simulink model "mpcLKAsystem"  (R2020b)
settings: Solver=VariableStepAuto  StartTime=0.0  StopTime=15  RelTol=1e-3
values from neighbouring files (symbols this model uses):
  Cf = 19000    [VehicleSteeringControlExample.m]
  Cr = 33000    [VehicleSteeringControlExample.m]
  Iz = 2875    [VehicleSteeringControlExample.m]
  lf = 1.2    [VehicleSteeringControlExample.m]
  lr = 1.6    [VehicleSteeringControlExample.m]
  m = 1575    [VehicleSteeringControlExample.m]
  md = getCurvature(Vx,time)    [VehicleSteeringControlExample.m]
  Ts = 0.1    [VehicleSteeringControlExample.m]
  Vx = 15    [VehicleSteeringControlExample.m]
libraries: mpcadaslib x1
settings Model: Creator=The MathWorks, Inc.  LastModifiedBy=j10
settings DataIOCC: ReturnWorkspaceOutputs=off
settings DebuggingCC: ArithmeticOperatorsInVariantConditions=warning
settings SFSimCC: SimUseLocalCustomCode=off  CustomCodeUndefinedFunction=UseInterfaceOnly
settings RTWCC: RTWUseLocalCustomCode=off
settings CodeAppCC: StateflowObjectComments=on
settings SimscapeCC: SimscapeNormalizeSystem=off

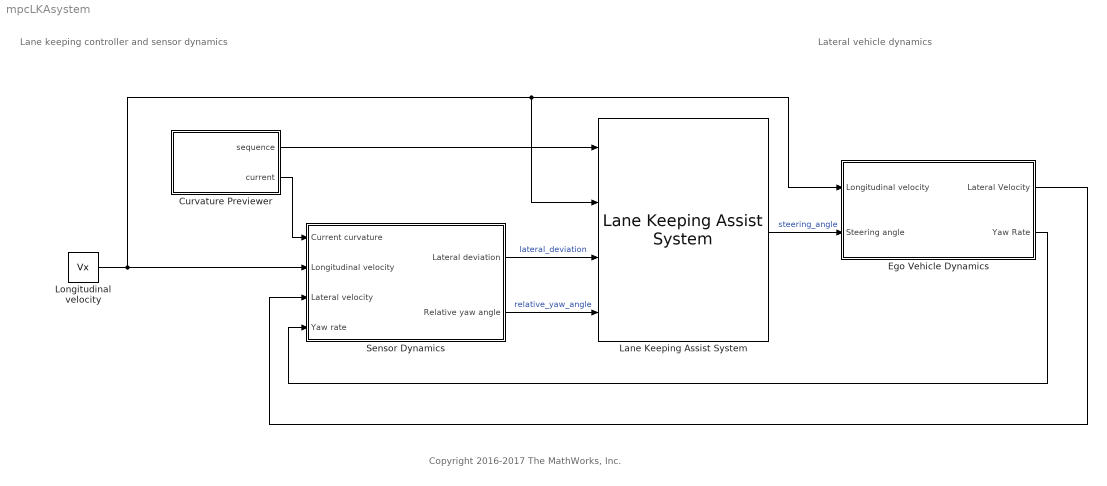
== system mpcLKAsystem ==
  note: Lateral vehicle dynamics
  note: Lane keeping controller and sensor dynamics
  note: Copyright 2016-2017 The MathWorks, Inc.
  Curvature Previewer : Subsystem  mask{signal=md, ts=Ts, steps=10}
      mask prompts: signal "Signal name"; ts "Sampling time"; steps "Number of previewing steps"
      mask init:
      | ts = evalin('base',get_param(gcbh,'ts'));
      | signal = evalin('base',get_param(gcbh,'signal'));
      | steps = evalin('base',get_param(gcbh,'steps'));
      | data = mpc_previewer_maskinit(signal,ts);
      mask Display:
      | fprintf('Future\nsample\nextractor');
      | port_label('output', 1, 'seq')
      | port_label('output', 2, '@t')
  Ego Vehicle Dynamics : Subsystem
  Lane Keeping Assist System : mpcadaslib/Lane Keeping Assist System  ModelType=Use vehicle parameters  VehicleMass=1575  VehicleYawInertia=2875  LengthToFront=1.2  LengthToRear=1.6  FrontTireStiffness=19000  RearTireStiffness=33000  EgoModelMatrixA=[-4.4021 ,-12.4603;1.3913,-5.1868]  EgoModelMatrixB=[24.1270;15.8609]  EgoModelMatrixC=[1,0;0,1]  InitialLongVel=15  TransportLag=0  MinSteering=-0.26  umin_ext=off  MaxSteering=0.26  umax_ext=off  Ts=0.1  PredictionHorizon=10  ControllerBehavior=0.5  suboptimal=off  maxiter=10  datatypeopt=double  optmode=off  trackmode=off
      settings: SourceProductBaseCode=MP
  Longitudinal velocity : Constant  Value=Vx  SampleTime=Ts
  Sensor Dynamics : Subsystem
  wires:
  Ego Vehicle Dynamics/2(Yaw Rate) -> Sensor Dynamics/4(Yaw rate)
  Ego Vehicle Dynamics/1(Lateral Velocity) -> Sensor Dynamics/3(Lateral velocity)
  Sensor Dynamics/1(Lateral deviation) -> Lane Keeping Assist System/3  "lateral_deviation"
  Sensor Dynamics/2(Relative yaw angle) -> Lane Keeping Assist System/4  "relative_yaw_angle"
  Longitudinal velocity/1 -> Lane Keeping Assist System/2, Ego Vehicle Dynamics/1(Longitudinal velocity), Sensor Dynamics/2(Longitudinal velocity)
  Curvature Previewer/1(sequence) -> Lane Keeping Assist System/1
  Lane Keeping Assist System/1 -> Ego Vehicle Dynamics/2(Steering angle)  "steering_angle"
  Curvature Previewer/2(current) -> Sensor Dynamics/1(Current curvature)

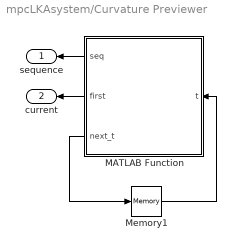
== system mpcLKAsystem/Curvature Previewer ==
  MATLAB Function : MATLAB Function  TreatAsAtomicUnit=on
  Memory1 : Memory  InheritSampleTime=on  LinearizeAsDelay=on
  sequence : Outport  VectorParamsAs1DForOutWhenUnconnected=off
  current : Outport  Port=2  VectorParamsAs1DForOutWhenUnconnected=off
  wires:
  MATLAB Function/1(seq) -> sequence/1
  MATLAB Function/2(first) -> current/1
  Memory1/1 -> MATLAB Function/1(t)
  MATLAB Function/3(next_t) -> Memory1/1

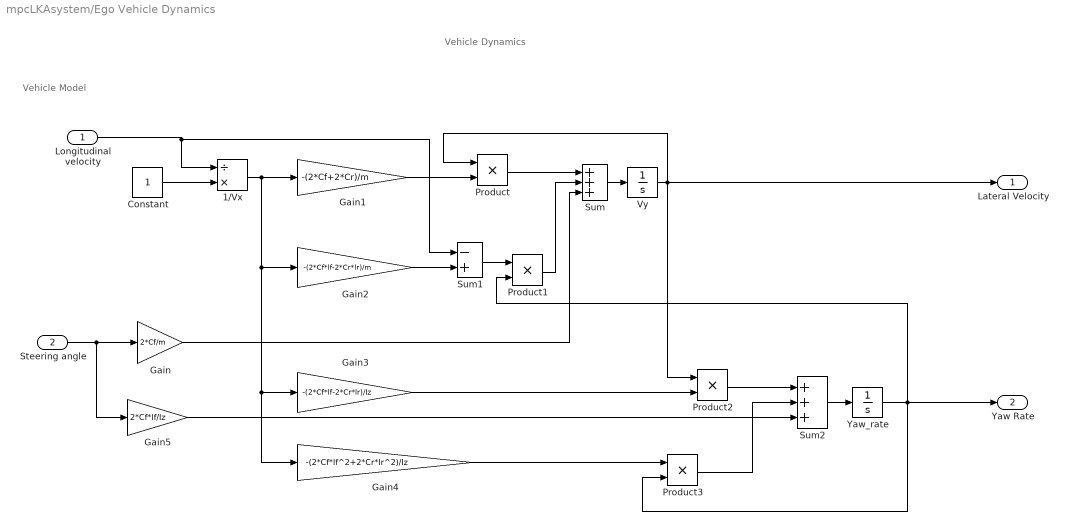
== system mpcLKAsystem/Ego Vehicle Dynamics ==
  note: Vehicle Model
  note: Vehicle Dynamics
  Longitudinal velocity : Inport
  Steering angle : Inport  Port=2
  1/Vx : Product  Inputs=/*
  Constant : Constant
  Gain : Gain  Gain=2*Cf/m
  Gain1 : Gain  Gain=-(2*Cf+2*Cr)/m
  Gain2 : Gain  Gain=-(2*Cf*lf-2*Cr*lr)/m
  Gain3 : Gain  Gain=-(2*Cf*lf-2*Cr*lr)/Iz
  Gain4 : Gain  Gain=-(2*Cf*lf^2+2*Cr*lr^2)/Iz
  Gain5 : Gain  Gain=2*Cf*lf/Iz
  Product{,1..3} (4 alike) : Product
  Sum : Sum  Inputs=+++
  Sum1 : Sum  Inputs=-+
  Sum2 : Sum  Inputs=+++
  Vy : Integrator
  "Yaw_rate " : Integrator
  Lateral Velocity : Outport  VectorParamsAs1DForOutWhenUnconnected=off
  Yaw Rate : Outport  Port=2  VectorParamsAs1DForOutWhenUnconnected=off
  wires:
  Sum2/1 -> "Yaw_rate "/1
  Gain2/1 -> Sum1/2
  Gain4/1 -> Product3/1
  Constant/1 -> 1/Vx/2
  Gain3/1 -> Product2/2
  1/Vx/1 -> Gain4/1, Gain3/1, Gain2/1, Gain1/1
  Product2/1 -> Sum2/1
  Product3/1 -> Sum2/2
  Gain5/1 -> Sum2/3
  Sum1/1 -> Product1/1
  "Yaw_rate "/1 -> Product3/2, Yaw Rate/1, Product1/2
  Gain/1 -> Sum/3
  Steering angle/1 -> Gain/1, Gain5/1
  Gain1/1 -> Product/2
  Product/1 -> Sum/1
  Vy/1 -> Product/1, Lateral Velocity/1, Product2/1
  Sum/1 -> Vy/1
  Longitudinal velocity/1 -> Sum1/1, 1/Vx/1
  Product1/1 -> Sum/2

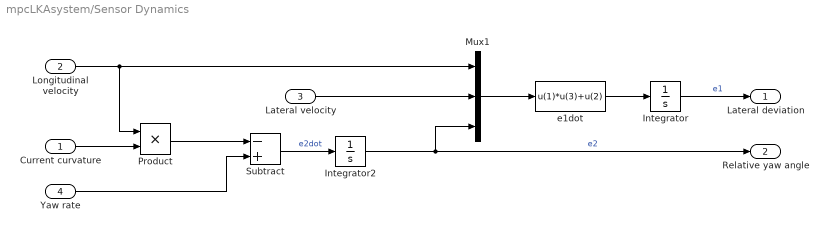
== system mpcLKAsystem/Sensor Dynamics ==
  Current curvature : Inport
  Longitudinal velocity : Inport  Port=2
  Lateral velocity : Inport  Port=3
  Yaw rate : Inport  Port=4
  Integrator : Integrator
  Integrator2 : Integrator
  Mux1 : Mux  Inputs=[1 1 1]
  Product : Product
  Subtract : Sum  Inputs=-+
  e1dot : Fcn  Expr=u(1)*u(3)+u(2)
  Lateral deviation : Outport  VectorParamsAs1DForOutWhenUnconnected=off
  Relative yaw angle : Outport  Port=2  VectorParamsAs1DForOutWhenUnconnected=off
  wires:
  Current curvature/1 -> Product/2
  Integrator2/1 -> Mux1/3, Relative yaw angle/1  "e2"
  Mux1/1 -> e1dot/1
  e1dot/1 -> Integrator/1
  Longitudinal velocity/1 -> Product/1, Mux1/1
  Lateral velocity/1 -> Mux1/2
  Integrator/1 -> Lateral deviation/1  "e1"
  Product/1 -> Subtract/1
  Yaw rate/1 -> Subtract/2
  Subtract/1 -> Integrator2/1  "e2dot"

== matlab function mpcLKAsystem/Curvature Previewer/MATLAB Function ==
  settings: updateMethod=DISCRETE  sampleTime=ts
  data: data parameter; seq output; steps parameter; t input; first output; next_t output
function [seq,first,next_t] = fcn(data,steps,t)
%#codegen
[seq,first,next_t] = mpcblock_preview('md',data,steps,t);
